simulink model "Cell"  (R2015a)
settings: Solver=ode45  StartTime=0.0  StopTime=10.0  RelTol=1e-3
model workspace (MAT data in the model file):
  Q0 = 0
values from neighbouring files (symbols this model uses):
  C1 = 404.263753891    [Samsung-25R.mat]
  Capacity = 2.5 * PACK_NUM_PARALLEL * 3600    (= 90000)    [Balancer_model_init.m]
  R1 = 0.00993116784096    [Samsung-25R.mat]
  Ri = 0.025    [Balancer_model_init.m]
  Voc =     [Samsung-25R.mat]
undefined symbols (not defined in the file or in its folder): Vc0
settings Model: ParameterArgumentNames=Q0  Creator=abk  LastModifiedBy=abk

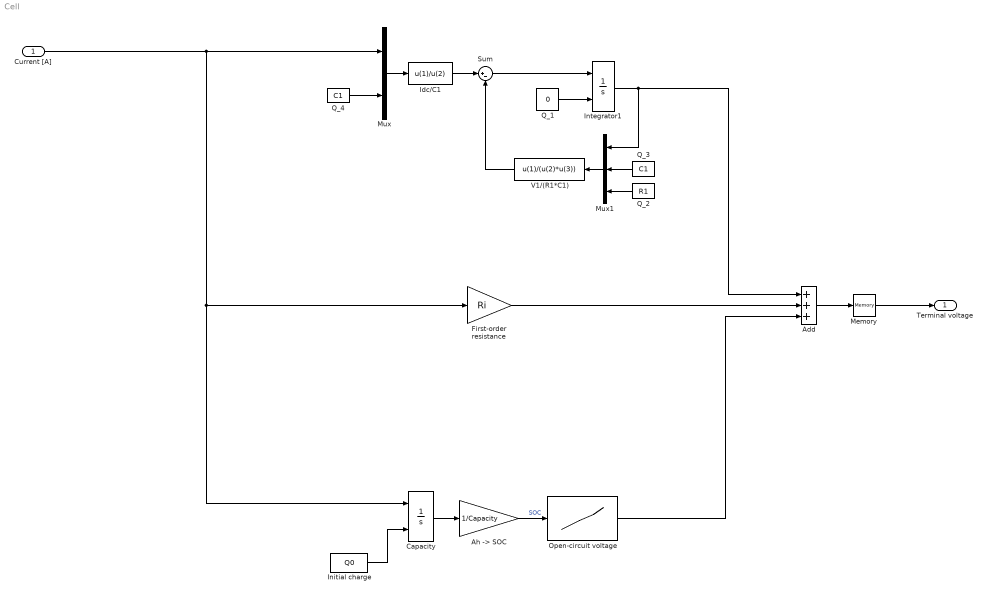
== system Cell ==
  Current [A] : Inport
  Add : Sum  Inputs=+++
  "Ah -> SOC" : Gain  Gain=1/Capacity
  Capacity : Integrator  InitialConditionSource=external  InitialCondition=Q0
  First-order resistance : Gain  Gain=Ri
  Idc/C1 : Fcn  Expr=u(1)/u(2)
  Initial charge : Constant  Value=Q0
  Integrator1 : Integrator  InitialConditionSource=external  InitialCondition=Vc0
  Memory : Memory
  Mux : Mux  Inputs=2
  Mux1 : Mux  Inputs=3
  Open-circuit voltage : Lookup_n-D  NumberOfTableDimensions=1  BreakpointsForDimension1=Voc.SOC  Table=Voc.V  InternalRulePriority=Speed  RndMeth=Simplest  InputSameDT=on
  Q_1 : Constant  Value=0
  Q_2 : Constant  Value=R1
  Q_3 : Constant  Value=C1
  Q_4 : Constant  Value=C1
  Sum : Sum  Inputs=|+-
  V1/(R1*C1) : Fcn  Expr=u(1)/(u(2)*u(3))
  Terminal voltage : Outport
  wires:
  "Ah -> SOC"/1 -> Open-circuit voltage/1  "SOC"
  Capacity/1 -> "Ah -> SOC"/1
  Initial charge/1 -> Capacity/2
  Add/1 -> Memory/1
  First-order resistance/1 -> Add/2
  Open-circuit voltage/1 -> Add/3
  Integrator1/1 -> Mux1/1, Add/1
  Current [A]/1 -> Capacity/1, First-order resistance/1, Mux/1
  Mux1/1 -> V1/(R1*C1)/1
  Mux/1 -> Idc/C1/1
  Sum/1 -> Integrator1/1
  Idc/C1/1 -> Sum/1
  V1/(R1*C1)/1 -> Sum/2
  Q_4/1 -> Mux/2
  Q_1/1 -> Integrator1/2
  Q_3/1 -> Mux1/2
  Q_2/1 -> Mux1/3
  Memory/1 -> Terminal voltage/1
